simulink model "Quadcopter_nonlinear"  (R2023a)
settings: Solver=ode4  StartTime=0.0  StopTime=0.2  FixedStep=0.02  RelTol=1e-3
values from neighbouring files (symbols this model uses):
  b = 1.10794e-5    (= 1.10794e-05)    [QuadParameter.m]
  d = 3.2e-6    (= 3.2e-06)    [QuadParameter.m]
  d_cg = 0.295    [QuadParameter.m]
  Gamma1 = 4.98954110218396e-06    (= 4.98954110218e-06)    [final_PS.m]
  Gamma10 = -1.44562619785504e-05    (= -1.44562619786e-05)    [final_PS.m]
  Gamma11 = 24.4566929368231    (= 24.4566929368)    [final_PS.m]
  Gamma2 = 0.00290613207976024    (= 0.00290613207976)    [final_PS.m]
  Gamma3 = 42.1805100768496    (= 42.1805100768)    [final_PS.m]
  Gamma4 = 0.000237183411278011    (= 0.000237183411278)    [final_PS.m]
  Gamma5 = -0.00234577516229748    (= -0.0023457751623)    [final_PS.m]
  Gamma6 = 2.52935414320957    (= 2.52935414321)    [final_PS.m]
  Gamma7 = 0.000224057181768728    (= 0.000224057181769)    [final_PS.m]
  Gamma8 = 18.4688604256806    (= 18.4688604257)    [final_PS.m]
  Gamma9 = 0.00216966508125569    (= 0.00216966508126)    [final_PS.m]
  init_I = data_I(1, :)    [PS_I.m]
  init_II = data_II(1, :)    [PS_II.m]
  init_III = data_III(1, :)    [PS_III.m]
  init_IV = data_IV(1, :)    [PS_IV.m]
  init_IX = data_IX(1, :)    [PS_IX.m]
  init_V = data_V(1, :)    [PS_V.m]
  init_VI = data_VI(1, :)    [PS_VI.m]
  Omega_I = Omega(1, :)    [PS_I.m]
  Omega_II = Omega(1, :)    [PS_II.m]
  Omega_III = Omega(1, :)    [PS_III.m]
  Omega_IV = Omega(1, :)    [PS_IV.m]
  Omega_IX = Omega(1, :)    [PS_IX.m]
  Omega_V = Omega(1, :)    [PS_V.m]
  Omega_VI = Omega(1, :)    [PS_VI.m]
  Omega_VII = Omega(1, :)    [PS_VII.m]
  Omega_VIII = Omega(1, :)    [PS_VIII.m]
  Omega_X = Omega(1, :)    [PS_X.m]
undefined symbols (not defined in the file or in its folder): init_VII, init_VIII, init_X
(part 3 of 3)

== system Quadcopter_nonlinear/Quadcopter 3DOF Nonlinear System8/Quad System1/Quad System/dot(x1)/Subsystem1 ==
  X : Inport
  Demux : Demux  Outputs=6
  Terminator{,2..5} (5 alike) : Terminator
  x4 : Outport
  wires:
  Demux/6 -> Terminator5/1  "x6"
  X/1 -> Demux/1
  Demux/3 -> Terminator/1  "x3"
  Demux/1 -> Terminator4/1  "x1"
  Demux/2 -> Terminator2/1  "x2"
  Demux/5 -> Terminator3/1  "x5"
  Demux/4 -> x4/1  "x4"

== system Quadcopter_nonlinear/Quadcopter 3DOF Nonlinear System8/Quad System1/Quad System/dot(x2)/1 ==
  X : Inport
  Demux : Demux  Outputs=6
  Subsystem : Subsystem
  Terminator{,1..3} (4 alike) : Terminator
  x5cos(x1) : Outport
  wires:
  Demux/4 -> Terminator1/1  "x4"
  X/1 -> Demux/1  "x"
  Demux/1 -> Subsystem/1(x1)  "x1"
  Demux/3 -> Terminator/1  "x3"
  Demux/6 -> Terminator2/1  "x6"
  Demux/5 -> Subsystem/2(x5)  "x5"
  Subsystem/1(Out1) -> x5cos(x1)/1
  Demux/2 -> Terminator3/1  "x2"

== system Quadcopter_nonlinear/Quadcopter 3DOF Nonlinear System8/Quad System1/Quad System/dot(x2)/Subsystem ==
  X : Inport
  Demux : Demux  Outputs=6
  Subsystem1 : Subsystem
  Terminator{,1..3} (4 alike) : Terminator
  x6sin(x1) : Outport
  wires:
  Demux/1 -> Subsystem1/1(x1)  "x1"
  Demux/3 -> Terminator/1  "x3"
  Demux/4 -> Terminator1/1  "x4"
  Demux/5 -> Terminator3/1  "x5"
  Demux/6 -> Subsystem1/2(x6)  "x6"
  Subsystem1/1(Out1) -> x6sin(x1)/1  "x6sin(x1)"
  X/1 -> Demux/1  "X"
  Demux/2 -> Terminator2/1  "x2"

== system Quadcopter_nonlinear/Quadcopter 3DOF Nonlinear System8/Quad System1/Quad System/dot(x3)/1 ==
  X : Inport
  Demux : Demux  Outputs=6
  Subsystem : Subsystem
  Terminator{,1..3} (4 alike) : Terminator
  x5sin(x1) : Outport
  wires:
  Demux/4 -> Terminator1/1  "x4"
  X/1 -> Demux/1  "x"
  Demux/1 -> Subsystem/1(x1)  "x1"
  Demux/3 -> Terminator/1  "x3"
  Demux/6 -> Terminator2/1  "x6"
  Demux/5 -> Subsystem/2(x5)  "x5"
  Subsystem/1(x5sin(x1)) -> x5sin(x1)/1
  Demux/2 -> Terminator3/1  "x2"

== system Quadcopter_nonlinear/Quadcopter 3DOF Nonlinear System8/Quad System1/Quad System/dot(x3)/Subsystem ==
  X : Inport
  Demux : Demux  Outputs=6
  Subsystem1 : Subsystem
  Terminator{,1..3} (4 alike) : Terminator
  x6cos(x1) : Outport
  wires:
  Demux/1 -> Subsystem1/1(x1)  "x1"
  Demux/3 -> Terminator/1  "x3"
  Demux/4 -> Terminator1/1  "x4"
  Demux/5 -> Terminator3/1  "x5"
  Demux/6 -> Subsystem1/2(x6)  "x6"
  Subsystem1/1(Out1) -> x6cos(x1)/1  "x6cos(x1)"
  X/1 -> Demux/1  "X"
  Demux/2 -> Terminator2/1  "x2"

== system Quadcopter_nonlinear/Quadcopter 3DOF Nonlinear System8/Quad System1/Quad System/dot(x3)/Subsystem1 ==
  X : Inport
  Demux : Demux  Outputs=6
  Sec : Subsystem
  Terminator{,1..4} (5 alike) : Terminator
  sec(x2) : Outport
  wires:
  Demux/3 -> Terminator/1  "x3"
  Demux/4 -> Terminator1/1  "x4"
  Demux/5 -> Terminator3/1  "x5"
  X/1 -> Demux/1  "X"
  Demux/1 -> Terminator2/1  "x1"
  Demux/6 -> Terminator4/1  "x6"
  Demux/2 -> Sec/1(x2)  "x2"
  Sec/1(Sec(x2)) -> sec(x2)/1

== system Quadcopter_nonlinear/Quadcopter 3DOF Nonlinear System9/Quad System1/Quad System/dot(x1)/1 ==
  X : Inport
  Demux : Demux  Outputs=6
  Subsystem : Subsystem
  Terminator : Terminator
  Terminator1 : Terminator
  Terminator2 : Terminator
  x5sin(x1)tan(x2) : Outport
  wires:
  Demux/2 -> Subsystem/2(x2)  "x2"
  Demux/4 -> Terminator1/1  "x4"
  X/1 -> Demux/1  "x"
  Demux/1 -> Subsystem/1(x1)  "x1"
  Demux/3 -> Terminator/1  "x3"
  Demux/6 -> Terminator2/1  "x6"
  Demux/5 -> Subsystem/3(x5)  "x5"
  Subsystem/1(x5sin(x1)tan(x2)) -> x5sin(x1)tan(x2)/1

== system Quadcopter_nonlinear/Quadcopter 3DOF Nonlinear System9/Quad System1/Quad System/dot(x1)/Subsystem ==
  X : Inport
  Demux : Demux  Outputs=6
  Subsystem1 : Subsystem
  Terminator : Terminator
  Terminator1 : Terminator
  Terminator3 : Terminator
  x6cos(x1)tan(x2) : Outport
  wires:
  Demux/1 -> Subsystem1/1(x1)  "x1"
  Demux/3 -> Terminator/1  "x3"
  Demux/4 -> Terminator1/1  "x4"
  Demux/5 -> Terminator3/1  "x5"
  Demux/6 -> Subsystem1/3(x6)  "x6"
  Subsystem1/1(x6cos(x1)tan(x2)) -> x6cos(x1)tan(x2)/1  "x6cos(x1)tan(x2)"
  X/1 -> Demux/1  "X"
  Demux/2 -> Subsystem1/2(x2)  "x2"

== system Quadcopter_nonlinear/Quadcopter 3DOF Nonlinear System9/Quad System1/Quad System/dot(x1)/Subsystem1 ==
  X : Inport
  Demux : Demux  Outputs=6
  Terminator{,2..5} (5 alike) : Terminator
  x4 : Outport
  wires:
  Demux/6 -> Terminator5/1  "x6"
  X/1 -> Demux/1
  Demux/3 -> Terminator/1  "x3"
  Demux/1 -> Terminator4/1  "x1"
  Demux/2 -> Terminator2/1  "x2"
  Demux/5 -> Terminator3/1  "x5"
  Demux/4 -> x4/1  "x4"

== system Quadcopter_nonlinear/Quadcopter 3DOF Nonlinear System9/Quad System1/Quad System/dot(x2)/1 ==
  X : Inport
  Demux : Demux  Outputs=6
  Subsystem : Subsystem
  Terminator{,1..3} (4 alike) : Terminator
  x5cos(x1) : Outport
  wires:
  Demux/4 -> Terminator1/1  "x4"
  X/1 -> Demux/1  "x"
  Demux/1 -> Subsystem/1(x1)  "x1"
  Demux/3 -> Terminator/1  "x3"
  Demux/6 -> Terminator2/1  "x6"
  Demux/5 -> Subsystem/2(x5)  "x5"
  Subsystem/1(Out1) -> x5cos(x1)/1
  Demux/2 -> Terminator3/1  "x2"

== system Quadcopter_nonlinear/Quadcopter 3DOF Nonlinear System9/Quad System1/Quad System/dot(x2)/Subsystem ==
  X : Inport
  Demux : Demux  Outputs=6
  Subsystem1 : Subsystem
  Terminator{,1..3} (4 alike) : Terminator
  x6sin(x1) : Outport
  wires:
  Demux/1 -> Subsystem1/1(x1)  "x1"
  Demux/3 -> Terminator/1  "x3"
  Demux/4 -> Terminator1/1  "x4"
  Demux/5 -> Terminator3/1  "x5"
  Demux/6 -> Subsystem1/2(x6)  "x6"
  Subsystem1/1(Out1) -> x6sin(x1)/1  "x6sin(x1)"
  X/1 -> Demux/1  "X"
  Demux/2 -> Terminator2/1  "x2"

== system Quadcopter_nonlinear/Quadcopter 3DOF Nonlinear System9/Quad System1/Quad System/dot(x3)/1 ==
  X : Inport
  Demux : Demux  Outputs=6
  Subsystem : Subsystem
  Terminator{,1..3} (4 alike) : Terminator
  x5sin(x1) : Outport
  wires:
  Demux/4 -> Terminator1/1  "x4"
  X/1 -> Demux/1  "x"
  Demux/1 -> Subsystem/1(x1)  "x1"
  Demux/3 -> Terminator/1  "x3"
  Demux/6 -> Terminator2/1  "x6"
  Demux/5 -> Subsystem/2(x5)  "x5"
  Subsystem/1(x5sin(x1)) -> x5sin(x1)/1
  Demux/2 -> Terminator3/1  "x2"

== system Quadcopter_nonlinear/Quadcopter 3DOF Nonlinear System9/Quad System1/Quad System/dot(x3)/Subsystem ==
  X : Inport
  Demux : Demux  Outputs=6
  Subsystem1 : Subsystem
  Terminator{,1..3} (4 alike) : Terminator
  x6cos(x1) : Outport
  wires:
  Demux/1 -> Subsystem1/1(x1)  "x1"
  Demux/3 -> Terminator/1  "x3"
  Demux/4 -> Terminator1/1  "x4"
  Demux/5 -> Terminator3/1  "x5"
  Demux/6 -> Subsystem1/2(x6)  "x6"
  Subsystem1/1(Out1) -> x6cos(x1)/1  "x6cos(x1)"
  X/1 -> Demux/1  "X"
  Demux/2 -> Terminator2/1  "x2"

== system Quadcopter_nonlinear/Quadcopter 3DOF Nonlinear System9/Quad System1/Quad System/dot(x3)/Subsystem1 ==
  X : Inport
  Demux : Demux  Outputs=6
  Sec : Subsystem
  Terminator{,1..4} (5 alike) : Terminator
  sec(x2) : Outport
  wires:
  Demux/3 -> Terminator/1  "x3"
  Demux/4 -> Terminator1/1  "x4"
  Demux/5 -> Terminator3/1  "x5"
  X/1 -> Demux/1  "X"
  Demux/1 -> Terminator2/1  "x1"
  Demux/6 -> Terminator4/1  "x6"
  Demux/2 -> Sec/1(x2)  "x2"
  Sec/1(Sec(x2)) -> sec(x2)/1

== system Quadcopter_nonlinear/Quadcopter 3DOF Nonlinear System/Quad System1/Quad System/dot(x1)/1/Subsystem ==
  x1 : Inport
  x2 : Inport  Port=2
  x5 : Inport  Port=3
  Product : Product  Inputs=3
  Sin : Trigonometry
  Tan : Trigonometry  Operator=tan
  x5sin(x1)tan(x2) : Outport
  wires:
  Sin/1 -> Product/1
  x5/1 -> Product/3
  Product/1 -> x5sin(x1)tan(x2)/1
  x1/1 -> Sin/1
  x2/1 -> Tan/1
  Tan/1 -> Product/2

== system Quadcopter_nonlinear/Quadcopter 3DOF Nonlinear System/Quad System1/Quad System/dot(x1)/Subsystem/Subsystem1 ==
  x1 : Inport
  x2 : Inport  Port=2
  x6 : Inport  Port=3
  Cos : Trigonometry  Operator=cos
  Product1 : Product  Inputs=3
  Tan : Trigonometry  Operator=tan
  x6cos(x1)tan(x2) : Outport
  wires:
  x6/1 -> Product1/3
  x1/1 -> Cos/1
  Cos/1 -> Product1/1
  x2/1 -> Tan/1
  Product1/1 -> x6cos(x1)tan(x2)/1
  Tan/1 -> Product1/2

== system Quadcopter_nonlinear/Quadcopter 3DOF Nonlinear System/Quad System1/Quad System/dot(x2)/1/Subsystem ==
  x1 : Inport
  x5 : Inport  Port=2
  Cos : Trigonometry  Operator=cos
  Product : Product
  Out1 : Outport
  wires:
  Cos/1 -> Product/1
  Product/1 -> Out1/1
  x1/1 -> Cos/1
  x5/1 -> Product/2

== system Quadcopter_nonlinear/Quadcopter 3DOF Nonlinear System/Quad System1/Quad System/dot(x2)/Subsystem/Subsystem1 ==
  x1 : Inport
  x6 : Inport  Port=2
  Product1 : Product
  Sin : Trigonometry
  Out1 : Outport
  wires:
  x6/1 -> Product1/2
  x1/1 -> Sin/1
  Sin/1 -> Product1/1
  Product1/1 -> Out1/1

== system Quadcopter_nonlinear/Quadcopter 3DOF Nonlinear System/Quad System1/Quad System/dot(x3)/1/Subsystem ==
  x1 : Inport
  x5 : Inport  Port=2
  Product : Product
  Sin : Trigonometry
  x5sin(x1) : Outport
  wires:
  Sin/1 -> Product/1
  Product/1 -> x5sin(x1)/1
  x1/1 -> Sin/1
  x5/1 -> Product/2

== system Quadcopter_nonlinear/Quadcopter 3DOF Nonlinear System/Quad System1/Quad System/dot(x3)/Subsystem/Subsystem1 ==
  x1 : Inport
  x6 : Inport  Port=2
  Cos : Trigonometry  Operator=cos
  Product1 : Product
  Out1 : Outport
  wires:
  x6/1 -> Product1/2
  x1/1 -> Cos/1
  Cos/1 -> Product1/1
  Product1/1 -> Out1/1

== system Quadcopter_nonlinear/Quadcopter 3DOF Nonlinear System/Quad System1/Quad System/dot(x3)/Subsystem1/Sec ==
  x2 : Inport
  Constant : Constant
  Cos : Trigonometry  Operator=cos
  Divide : Product  Inputs=*/
  Sec(x2) : Outport
  wires:
  Constant/1 -> Divide/1
  Cos/1 -> Divide/2
  Divide/1 -> Sec(x2)/1
  x2/1 -> Cos/1

== system Quadcopter_nonlinear/Quadcopter 3DOF Nonlinear System1/Quad System1/Quad System/dot(x1)/1/Subsystem ==
  x1 : Inport
  x2 : Inport  Port=2
  x5 : Inport  Port=3
  Product : Product  Inputs=3
  Sin : Trigonometry
  Tan : Trigonometry  Operator=tan
  x5sin(x1)tan(x2) : Outport
  wires:
  Sin/1 -> Product/1
  x5/1 -> Product/3
  Product/1 -> x5sin(x1)tan(x2)/1
  x1/1 -> Sin/1
  x2/1 -> Tan/1
  Tan/1 -> Product/2

== system Quadcopter_nonlinear/Quadcopter 3DOF Nonlinear System1/Quad System1/Quad System/dot(x1)/Subsystem/Subsystem1 ==
  x1 : Inport
  x2 : Inport  Port=2
  x6 : Inport  Port=3
  Cos : Trigonometry  Operator=cos
  Product1 : Product  Inputs=3
  Tan : Trigonometry  Operator=tan
  x6cos(x1)tan(x2) : Outport
  wires:
  x6/1 -> Product1/3
  x1/1 -> Cos/1
  Cos/1 -> Product1/1
  x2/1 -> Tan/1
  Product1/1 -> x6cos(x1)tan(x2)/1
  Tan/1 -> Product1/2

== system Quadcopter_nonlinear/Quadcopter 3DOF Nonlinear System1/Quad System1/Quad System/dot(x2)/1/Subsystem ==
  x1 : Inport
  x5 : Inport  Port=2
  Cos : Trigonometry  Operator=cos
  Product : Product
  Out1 : Outport
  wires:
  Cos/1 -> Product/1
  Product/1 -> Out1/1
  x1/1 -> Cos/1
  x5/1 -> Product/2

== system Quadcopter_nonlinear/Quadcopter 3DOF Nonlinear System1/Quad System1/Quad System/dot(x2)/Subsystem/Subsystem1 ==
  x1 : Inport
  x6 : Inport  Port=2
  Product1 : Product
  Sin : Trigonometry
  Out1 : Outport
  wires:
  x6/1 -> Product1/2
  x1/1 -> Sin/1
  Sin/1 -> Product1/1
  Product1/1 -> Out1/1

== system Quadcopter_nonlinear/Quadcopter 3DOF Nonlinear System1/Quad System1/Quad System/dot(x3)/1/Subsystem ==
  x1 : Inport
  x5 : Inport  Port=2
  Product : Product
  Sin : Trigonometry
  x5sin(x1) : Outport
  wires:
  Sin/1 -> Product/1
  Product/1 -> x5sin(x1)/1
  x1/1 -> Sin/1
  x5/1 -> Product/2

== system Quadcopter_nonlinear/Quadcopter 3DOF Nonlinear System1/Quad System1/Quad System/dot(x3)/Subsystem/Subsystem1 ==
  x1 : Inport
  x6 : Inport  Port=2
  Cos : Trigonometry  Operator=cos
  Product1 : Product
  Out1 : Outport
  wires:
  x6/1 -> Product1/2
  x1/1 -> Cos/1
  Cos/1 -> Product1/1
  Product1/1 -> Out1/1

== system Quadcopter_nonlinear/Quadcopter 3DOF Nonlinear System1/Quad System1/Quad System/dot(x3)/Subsystem1/Sec ==
  x2 : Inport
  Constant : Constant
  Cos : Trigonometry  Operator=cos
  Divide : Product  Inputs=*/
  Sec(x2) : Outport
  wires:
  Constant/1 -> Divide/1
  Cos/1 -> Divide/2
  Divide/1 -> Sec(x2)/1
  x2/1 -> Cos/1

== system Quadcopter_nonlinear/Quadcopter 3DOF Nonlinear System2/Quad System1/Quad System/dot(x1)/1/Subsystem ==
  x1 : Inport
  x2 : Inport  Port=2
  x5 : Inport  Port=3
  Product : Product  Inputs=3
  Sin : Trigonometry
  Tan : Trigonometry  Operator=tan
  x5sin(x1)tan(x2) : Outport
  wires:
  Sin/1 -> Product/1
  x5/1 -> Product/3
  Product/1 -> x5sin(x1)tan(x2)/1
  x1/1 -> Sin/1
  x2/1 -> Tan/1
  Tan/1 -> Product/2

== system Quadcopter_nonlinear/Quadcopter 3DOF Nonlinear System2/Quad System1/Quad System/dot(x1)/Subsystem/Subsystem1 ==
  x1 : Inport
  x2 : Inport  Port=2
  x6 : Inport  Port=3
  Cos : Trigonometry  Operator=cos
  Product1 : Product  Inputs=3
  Tan : Trigonometry  Operator=tan
  x6cos(x1)tan(x2) : Outport
  wires:
  x6/1 -> Product1/3
  x1/1 -> Cos/1
  Cos/1 -> Product1/1
  x2/1 -> Tan/1
  Product1/1 -> x6cos(x1)tan(x2)/1
  Tan/1 -> Product1/2

== system Quadcopter_nonlinear/Quadcopter 3DOF Nonlinear System2/Quad System1/Quad System/dot(x2)/1/Subsystem ==
  x1 : Inport
  x5 : Inport  Port=2
  Cos : Trigonometry  Operator=cos
  Product : Product
  Out1 : Outport
  wires:
  Cos/1 -> Product/1
  Product/1 -> Out1/1
  x1/1 -> Cos/1
  x5/1 -> Product/2

== system Quadcopter_nonlinear/Quadcopter 3DOF Nonlinear System2/Quad System1/Quad System/dot(x2)/Subsystem/Subsystem1 ==
  x1 : Inport
  x6 : Inport  Port=2
  Product1 : Product
  Sin : Trigonometry
  Out1 : Outport
  wires:
  x6/1 -> Product1/2
  x1/1 -> Sin/1
  Sin/1 -> Product1/1
  Product1/1 -> Out1/1

== system Quadcopter_nonlinear/Quadcopter 3DOF Nonlinear System2/Quad System1/Quad System/dot(x3)/1/Subsystem ==
  x1 : Inport
  x5 : Inport  Port=2
  Product : Product
  Sin : Trigonometry
  x5sin(x1) : Outport
  wires:
  Sin/1 -> Product/1
  Product/1 -> x5sin(x1)/1
  x1/1 -> Sin/1
  x5/1 -> Product/2

== system Quadcopter_nonlinear/Quadcopter 3DOF Nonlinear System2/Quad System1/Quad System/dot(x3)/Subsystem/Subsystem1 ==
  x1 : Inport
  x6 : Inport  Port=2
  Cos : Trigonometry  Operator=cos
  Product1 : Product
  Out1 : Outport
  wires:
  x6/1 -> Product1/2
  x1/1 -> Cos/1
  Cos/1 -> Product1/1
  Product1/1 -> Out1/1

== system Quadcopter_nonlinear/Quadcopter 3DOF Nonlinear System2/Quad System1/Quad System/dot(x3)/Subsystem1/Sec ==
  x2 : Inport
  Constant : Constant
  Cos : Trigonometry  Operator=cos
  Divide : Product  Inputs=*/
  Sec(x2) : Outport
  wires:
  Constant/1 -> Divide/1
  Cos/1 -> Divide/2
  Divide/1 -> Sec(x2)/1
  x2/1 -> Cos/1

== system Quadcopter_nonlinear/Quadcopter 3DOF Nonlinear System3/Quad System1/Quad System/dot(x1)/1/Subsystem ==
  x1 : Inport
  x2 : Inport  Port=2
  x5 : Inport  Port=3
  Product : Product  Inputs=3
  Sin : Trigonometry
  Tan : Trigonometry  Operator=tan
  x5sin(x1)tan(x2) : Outport
  wires:
  Sin/1 -> Product/1
  x5/1 -> Product/3
  Product/1 -> x5sin(x1)tan(x2)/1
  x1/1 -> Sin/1
  x2/1 -> Tan/1
  Tan/1 -> Product/2

== system Quadcopter_nonlinear/Quadcopter 3DOF Nonlinear System3/Quad System1/Quad System/dot(x1)/Subsystem/Subsystem1 ==
  x1 : Inport
  x2 : Inport  Port=2
  x6 : Inport  Port=3
  Cos : Trigonometry  Operator=cos
  Product1 : Product  Inputs=3
  Tan : Trigonometry  Operator=tan
  x6cos(x1)tan(x2) : Outport
  wires:
  x6/1 -> Product1/3
  x1/1 -> Cos/1
  Cos/1 -> Product1/1
  x2/1 -> Tan/1
  Product1/1 -> x6cos(x1)tan(x2)/1
  Tan/1 -> Product1/2

== system Quadcopter_nonlinear/Quadcopter 3DOF Nonlinear System3/Quad System1/Quad System/dot(x2)/1/Subsystem ==
  x1 : Inport
  x5 : Inport  Port=2
  Cos : Trigonometry  Operator=cos
  Product : Product
  Out1 : Outport
  wires:
  Cos/1 -> Product/1
  Product/1 -> Out1/1
  x1/1 -> Cos/1
  x5/1 -> Product/2

== system Quadcopter_nonlinear/Quadcopter 3DOF Nonlinear System3/Quad System1/Quad System/dot(x2)/Subsystem/Subsystem1 ==
  x1 : Inport
  x6 : Inport  Port=2
  Product1 : Product
  Sin : Trigonometry
  Out1 : Outport
  wires:
  x6/1 -> Product1/2
  x1/1 -> Sin/1
  Sin/1 -> Product1/1
  Product1/1 -> Out1/1

== system Quadcopter_nonlinear/Quadcopter 3DOF Nonlinear System3/Quad System1/Quad System/dot(x3)/1/Subsystem ==
  x1 : Inport
  x5 : Inport  Port=2
  Product : Product
  Sin : Trigonometry
  x5sin(x1) : Outport
  wires:
  Sin/1 -> Product/1
  Product/1 -> x5sin(x1)/1
  x1/1 -> Sin/1
  x5/1 -> Product/2

== system Quadcopter_nonlinear/Quadcopter 3DOF Nonlinear System3/Quad System1/Quad System/dot(x3)/Subsystem/Subsystem1 ==
  x1 : Inport
  x6 : Inport  Port=2
  Cos : Trigonometry  Operator=cos
  Product1 : Product
  Out1 : Outport
  wires:
  x6/1 -> Product1/2
  x1/1 -> Cos/1
  Cos/1 -> Product1/1
  Product1/1 -> Out1/1

== system Quadcopter_nonlinear/Quadcopter 3DOF Nonlinear System3/Quad System1/Quad System/dot(x3)/Subsystem1/Sec ==
  x2 : Inport
  Constant : Constant
  Cos : Trigonometry  Operator=cos
  Divide : Product  Inputs=*/
  Sec(x2) : Outport
  wires:
  Constant/1 -> Divide/1
  Cos/1 -> Divide/2
  Divide/1 -> Sec(x2)/1
  x2/1 -> Cos/1

== system Quadcopter_nonlinear/Quadcopter 3DOF Nonlinear System4/Quad System1/Quad System/dot(x1)/1/Subsystem ==
  x1 : Inport
  x2 : Inport  Port=2
  x5 : Inport  Port=3
  Product : Product  Inputs=3
  Sin : Trigonometry
  Tan : Trigonometry  Operator=tan
  x5sin(x1)tan(x2) : Outport
  wires:
  Sin/1 -> Product/1
  x5/1 -> Product/3
  Product/1 -> x5sin(x1)tan(x2)/1
  x1/1 -> Sin/1
  x2/1 -> Tan/1
  Tan/1 -> Product/2

== system Quadcopter_nonlinear/Quadcopter 3DOF Nonlinear System4/Quad System1/Quad System/dot(x1)/Subsystem/Subsystem1 ==
  x1 : Inport
  x2 : Inport  Port=2
  x6 : Inport  Port=3
  Cos : Trigonometry  Operator=cos
  Product1 : Product  Inputs=3
  Tan : Trigonometry  Operator=tan
  x6cos(x1)tan(x2) : Outport
  wires:
  x6/1 -> Product1/3
  x1/1 -> Cos/1
  Cos/1 -> Product1/1
  x2/1 -> Tan/1
  Product1/1 -> x6cos(x1)tan(x2)/1
  Tan/1 -> Product1/2

== system Quadcopter_nonlinear/Quadcopter 3DOF Nonlinear System4/Quad System1/Quad System/dot(x2)/1/Subsystem ==
  x1 : Inport
  x5 : Inport  Port=2
  Cos : Trigonometry  Operator=cos
  Product : Product
  Out1 : Outport
  wires:
  Cos/1 -> Product/1
  Product/1 -> Out1/1
  x1/1 -> Cos/1
  x5/1 -> Product/2

== system Quadcopter_nonlinear/Quadcopter 3DOF Nonlinear System4/Quad System1/Quad System/dot(x2)/Subsystem/Subsystem1 ==
  x1 : Inport
  x6 : Inport  Port=2
  Product1 : Product
  Sin : Trigonometry
  Out1 : Outport
  wires:
  x6/1 -> Product1/2
  x1/1 -> Sin/1
  Sin/1 -> Product1/1
  Product1/1 -> Out1/1

== system Quadcopter_nonlinear/Quadcopter 3DOF Nonlinear System4/Quad System1/Quad System/dot(x3)/1/Subsystem ==
  x1 : Inport
  x5 : Inport  Port=2
  Product : Product
  Sin : Trigonometry
  x5sin(x1) : Outport
  wires:
  Sin/1 -> Product/1
  Product/1 -> x5sin(x1)/1
  x1/1 -> Sin/1
  x5/1 -> Product/2

== system Quadcopter_nonlinear/Quadcopter 3DOF Nonlinear System4/Quad System1/Quad System/dot(x3)/Subsystem/Subsystem1 ==
  x1 : Inport
  x6 : Inport  Port=2
  Cos : Trigonometry  Operator=cos
  Product1 : Product
  Out1 : Outport
  wires:
  x6/1 -> Product1/2
  x1/1 -> Cos/1
  Cos/1 -> Product1/1
  Product1/1 -> Out1/1

== system Quadcopter_nonlinear/Quadcopter 3DOF Nonlinear System4/Quad System1/Quad System/dot(x3)/Subsystem1/Sec ==
  x2 : Inport
  Constant : Constant
  Cos : Trigonometry  Operator=cos
  Divide : Product  Inputs=*/
  Sec(x2) : Outport
  wires:
  Constant/1 -> Divide/1
  Cos/1 -> Divide/2
  Divide/1 -> Sec(x2)/1
  x2/1 -> Cos/1

== system Quadcopter_nonlinear/Quadcopter 3DOF Nonlinear System5/Quad System1/Quad System/dot(x1)/1/Subsystem ==
  x1 : Inport
  x2 : Inport  Port=2
  x5 : Inport  Port=3
  Product : Product  Inputs=3
  Sin : Trigonometry
  Tan : Trigonometry  Operator=tan
  x5sin(x1)tan(x2) : Outport
  wires:
  Sin/1 -> Product/1
  x5/1 -> Product/3
  Product/1 -> x5sin(x1)tan(x2)/1
  x1/1 -> Sin/1
  x2/1 -> Tan/1
  Tan/1 -> Product/2

== system Quadcopter_nonlinear/Quadcopter 3DOF Nonlinear System5/Quad System1/Quad System/dot(x1)/Subsystem/Subsystem1 ==
  x1 : Inport
  x2 : Inport  Port=2
  x6 : Inport  Port=3
  Cos : Trigonometry  Operator=cos
  Product1 : Product  Inputs=3
  Tan : Trigonometry  Operator=tan
  x6cos(x1)tan(x2) : Outport
  wires:
  x6/1 -> Product1/3
  x1/1 -> Cos/1
  Cos/1 -> Product1/1
  x2/1 -> Tan/1
  Product1/1 -> x6cos(x1)tan(x2)/1
  Tan/1 -> Product1/2

== system Quadcopter_nonlinear/Quadcopter 3DOF Nonlinear System5/Quad System1/Quad System/dot(x2)/1/Subsystem ==
  x1 : Inport
  x5 : Inport  Port=2
  Cos : Trigonometry  Operator=cos
  Product : Product
  Out1 : Outport
  wires:
  Cos/1 -> Product/1
  Product/1 -> Out1/1
  x1/1 -> Cos/1
  x5/1 -> Product/2

== system Quadcopter_nonlinear/Quadcopter 3DOF Nonlinear System5/Quad System1/Quad System/dot(x2)/Subsystem/Subsystem1 ==
  x1 : Inport
  x6 : Inport  Port=2
  Product1 : Product
  Sin : Trigonometry
  Out1 : Outport
  wires:
  x6/1 -> Product1/2
  x1/1 -> Sin/1
  Sin/1 -> Product1/1
  Product1/1 -> Out1/1

== system Quadcopter_nonlinear/Quadcopter 3DOF Nonlinear System5/Quad System1/Quad System/dot(x3)/1/Subsystem ==
  x1 : Inport
  x5 : Inport  Port=2
  Product : Product
  Sin : Trigonometry
  x5sin(x1) : Outport
  wires:
  Sin/1 -> Product/1
  Product/1 -> x5sin(x1)/1
  x1/1 -> Sin/1
  x5/1 -> Product/2

== system Quadcopter_nonlinear/Quadcopter 3DOF Nonlinear System5/Quad System1/Quad System/dot(x3)/Subsystem/Subsystem1 ==
  x1 : Inport
  x6 : Inport  Port=2
  Cos : Trigonometry  Operator=cos
  Product1 : Product
  Out1 : Outport
  wires:
  x6/1 -> Product1/2
  x1/1 -> Cos/1
  Cos/1 -> Product1/1
  Product1/1 -> Out1/1

== system Quadcopter_nonlinear/Quadcopter 3DOF Nonlinear System5/Quad System1/Quad System/dot(x3)/Subsystem1/Sec ==
  x2 : Inport
  Constant : Constant
  Cos : Trigonometry  Operator=cos
  Divide : Product  Inputs=*/
  Sec(x2) : Outport
  wires:
  Constant/1 -> Divide/1
  Cos/1 -> Divide/2
  Divide/1 -> Sec(x2)/1
  x2/1 -> Cos/1

== system Quadcopter_nonlinear/Quadcopter 3DOF Nonlinear System6/Quad System1/Quad System/dot(x1)/1/Subsystem ==
  x1 : Inport
  x2 : Inport  Port=2
  x5 : Inport  Port=3
  Product : Product  Inputs=3
  Sin : Trigonometry
  Tan : Trigonometry  Operator=tan
  x5sin(x1)tan(x2) : Outport
  wires:
  Sin/1 -> Product/1
  x5/1 -> Product/3
  Product/1 -> x5sin(x1)tan(x2)/1
  x1/1 -> Sin/1
  x2/1 -> Tan/1
  Tan/1 -> Product/2

== system Quadcopter_nonlinear/Quadcopter 3DOF Nonlinear System6/Quad System1/Quad System/dot(x1)/Subsystem/Subsystem1 ==
  x1 : Inport
  x2 : Inport  Port=2
  x6 : Inport  Port=3
  Cos : Trigonometry  Operator=cos
  Product1 : Product  Inputs=3
  Tan : Trigonometry  Operator=tan
  x6cos(x1)tan(x2) : Outport
  wires:
  x6/1 -> Product1/3
  x1/1 -> Cos/1
  Cos/1 -> Product1/1
  x2/1 -> Tan/1
  Product1/1 -> x6cos(x1)tan(x2)/1
  Tan/1 -> Product1/2

== system Quadcopter_nonlinear/Quadcopter 3DOF Nonlinear System6/Quad System1/Quad System/dot(x2)/1/Subsystem ==
  x1 : Inport
  x5 : Inport  Port=2
  Cos : Trigonometry  Operator=cos
  Product : Product
  Out1 : Outport
  wires:
  Cos/1 -> Product/1
  Product/1 -> Out1/1
  x1/1 -> Cos/1
  x5/1 -> Product/2

== system Quadcopter_nonlinear/Quadcopter 3DOF Nonlinear System6/Quad System1/Quad System/dot(x2)/Subsystem/Subsystem1 ==
  x1 : Inport
  x6 : Inport  Port=2
  Product1 : Product
  Sin : Trigonometry
  Out1 : Outport
  wires:
  x6/1 -> Product1/2
  x1/1 -> Sin/1
  Sin/1 -> Product1/1
  Product1/1 -> Out1/1

== system Quadcopter_nonlinear/Quadcopter 3DOF Nonlinear System6/Quad System1/Quad System/dot(x3)/1/Subsystem ==
  x1 : Inport
  x5 : Inport  Port=2
  Product : Product
  Sin : Trigonometry
  x5sin(x1) : Outport
  wires:
  Sin/1 -> Product/1
  Product/1 -> x5sin(x1)/1
  x1/1 -> Sin/1
  x5/1 -> Product/2

== system Quadcopter_nonlinear/Quadcopter 3DOF Nonlinear System6/Quad System1/Quad System/dot(x3)/Subsystem/Subsystem1 ==
  x1 : Inport
  x6 : Inport  Port=2
  Cos : Trigonometry  Operator=cos
  Product1 : Product
  Out1 : Outport
  wires:
  x6/1 -> Product1/2
  x1/1 -> Cos/1
  Cos/1 -> Product1/1
  Product1/1 -> Out1/1

== system Quadcopter_nonlinear/Quadcopter 3DOF Nonlinear System6/Quad System1/Quad System/dot(x3)/Subsystem1/Sec ==
  x2 : Inport
  Constant : Constant
  Cos : Trigonometry  Operator=cos
  Divide : Product  Inputs=*/
  Sec(x2) : Outport
  wires:
  Constant/1 -> Divide/1
  Cos/1 -> Divide/2
  Divide/1 -> Sec(x2)/1
  x2/1 -> Cos/1

== system Quadcopter_nonlinear/Quadcopter 3DOF Nonlinear System7/Quad System1/Quad System/dot(x1)/1/Subsystem ==
  x1 : Inport
  x2 : Inport  Port=2
  x5 : Inport  Port=3
  Product : Product  Inputs=3
  Sin : Trigonometry
  Tan : Trigonometry  Operator=tan
  x5sin(x1)tan(x2) : Outport
  wires:
  Sin/1 -> Product/1
  x5/1 -> Product/3
  Product/1 -> x5sin(x1)tan(x2)/1
  x1/1 -> Sin/1
  x2/1 -> Tan/1
  Tan/1 -> Product/2

== system Quadcopter_nonlinear/Quadcopter 3DOF Nonlinear System7/Quad System1/Quad System/dot(x1)/Subsystem/Subsystem1 ==
  x1 : Inport
  x2 : Inport  Port=2
  x6 : Inport  Port=3
  Cos : Trigonometry  Operator=cos
  Product1 : Product  Inputs=3
  Tan : Trigonometry  Operator=tan
  x6cos(x1)tan(x2) : Outport
  wires:
  x6/1 -> Product1/3
  x1/1 -> Cos/1
  Cos/1 -> Product1/1
  x2/1 -> Tan/1
  Product1/1 -> x6cos(x1)tan(x2)/1
  Tan/1 -> Product1/2

== system Quadcopter_nonlinear/Quadcopter 3DOF Nonlinear System7/Quad System1/Quad System/dot(x2)/1/Subsystem ==
  x1 : Inport
  x5 : Inport  Port=2
  Cos : Trigonometry  Operator=cos
  Product : Product
  Out1 : Outport
  wires:
  Cos/1 -> Product/1
  Product/1 -> Out1/1
  x1/1 -> Cos/1
  x5/1 -> Product/2

== system Quadcopter_nonlinear/Quadcopter 3DOF Nonlinear System7/Quad System1/Quad System/dot(x2)/Subsystem/Subsystem1 ==
  x1 : Inport
  x6 : Inport  Port=2
  Product1 : Product
  Sin : Trigonometry
  Out1 : Outport
  wires:
  x6/1 -> Product1/2
  x1/1 -> Sin/1
  Sin/1 -> Product1/1
  Product1/1 -> Out1/1

== system Quadcopter_nonlinear/Quadcopter 3DOF Nonlinear System7/Quad System1/Quad System/dot(x3)/1/Subsystem ==
  x1 : Inport
  x5 : Inport  Port=2
  Product : Product
  Sin : Trigonometry
  x5sin(x1) : Outport
  wires:
  Sin/1 -> Product/1
  Product/1 -> x5sin(x1)/1
  x1/1 -> Sin/1
  x5/1 -> Product/2

== system Quadcopter_nonlinear/Quadcopter 3DOF Nonlinear System7/Quad System1/Quad System/dot(x3)/Subsystem/Subsystem1 ==
  x1 : Inport
  x6 : Inport  Port=2
  Cos : Trigonometry  Operator=cos
  Product1 : Product
  Out1 : Outport
  wires:
  x6/1 -> Product1/2
  x1/1 -> Cos/1
  Cos/1 -> Product1/1
  Product1/1 -> Out1/1

== system Quadcopter_nonlinear/Quadcopter 3DOF Nonlinear System7/Quad System1/Quad System/dot(x3)/Subsystem1/Sec ==
  x2 : Inport
  Constant : Constant
  Cos : Trigonometry  Operator=cos
  Divide : Product  Inputs=*/
  Sec(x2) : Outport
  wires:
  Constant/1 -> Divide/1
  Cos/1 -> Divide/2
  Divide/1 -> Sec(x2)/1
  x2/1 -> Cos/1

== system Quadcopter_nonlinear/Quadcopter 3DOF Nonlinear System8/Quad System1/Quad System/dot(x1)/1/Subsystem ==
  x1 : Inport
  x2 : Inport  Port=2
  x5 : Inport  Port=3
  Product : Product  Inputs=3
  Sin : Trigonometry
  Tan : Trigonometry  Operator=tan
  x5sin(x1)tan(x2) : Outport
  wires:
  Sin/1 -> Product/1
  x5/1 -> Product/3
  Product/1 -> x5sin(x1)tan(x2)/1
  x1/1 -> Sin/1
  x2/1 -> Tan/1
  Tan/1 -> Product/2

== system Quadcopter_nonlinear/Quadcopter 3DOF Nonlinear System8/Quad System1/Quad System/dot(x1)/Subsystem/Subsystem1 ==
  x1 : Inport
  x2 : Inport  Port=2
  x6 : Inport  Port=3
  Cos : Trigonometry  Operator=cos
  Product1 : Product  Inputs=3
  Tan : Trigonometry  Operator=tan
  x6cos(x1)tan(x2) : Outport
  wires:
  x6/1 -> Product1/3
  x1/1 -> Cos/1
  Cos/1 -> Product1/1
  x2/1 -> Tan/1
  Product1/1 -> x6cos(x1)tan(x2)/1
  Tan/1 -> Product1/2

== system Quadcopter_nonlinear/Quadcopter 3DOF Nonlinear System8/Quad System1/Quad System/dot(x2)/1/Subsystem ==
  x1 : Inport
  x5 : Inport  Port=2
  Cos : Trigonometry  Operator=cos
  Product : Product
  Out1 : Outport
  wires:
  Cos/1 -> Product/1
  Product/1 -> Out1/1
  x1/1 -> Cos/1
  x5/1 -> Product/2

== system Quadcopter_nonlinear/Quadcopter 3DOF Nonlinear System8/Quad System1/Quad System/dot(x2)/Subsystem/Subsystem1 ==
  x1 : Inport
  x6 : Inport  Port=2
  Product1 : Product
  Sin : Trigonometry
  Out1 : Outport
  wires:
  x6/1 -> Product1/2
  x1/1 -> Sin/1
  Sin/1 -> Product1/1
  Product1/1 -> Out1/1

== system Quadcopter_nonlinear/Quadcopter 3DOF Nonlinear System8/Quad System1/Quad System/dot(x3)/1/Subsystem ==
  x1 : Inport
  x5 : Inport  Port=2
  Product : Product
  Sin : Trigonometry
  x5sin(x1) : Outport
  wires:
  Sin/1 -> Product/1
  Product/1 -> x5sin(x1)/1
  x1/1 -> Sin/1
  x5/1 -> Product/2

== system Quadcopter_nonlinear/Quadcopter 3DOF Nonlinear System8/Quad System1/Quad System/dot(x3)/Subsystem/Subsystem1 ==
  x1 : Inport
  x6 : Inport  Port=2
  Cos : Trigonometry  Operator=cos
  Product1 : Product
  Out1 : Outport
  wires:
  x6/1 -> Product1/2
  x1/1 -> Cos/1
  Cos/1 -> Product1/1
  Product1/1 -> Out1/1

== system Quadcopter_nonlinear/Quadcopter 3DOF Nonlinear System8/Quad System1/Quad System/dot(x3)/Subsystem1/Sec ==
  x2 : Inport
  Constant : Constant
  Cos : Trigonometry  Operator=cos
  Divide : Product  Inputs=*/
  Sec(x2) : Outport
  wires:
  Constant/1 -> Divide/1
  Cos/1 -> Divide/2
  Divide/1 -> Sec(x2)/1
  x2/1 -> Cos/1

== system Quadcopter_nonlinear/Quadcopter 3DOF Nonlinear System9/Quad System1/Quad System/dot(x1)/1/Subsystem ==
  x1 : Inport
  x2 : Inport  Port=2
  x5 : Inport  Port=3
  Product : Product  Inputs=3
  Sin : Trigonometry
  Tan : Trigonometry  Operator=tan
  x5sin(x1)tan(x2) : Outport
  wires:
  Sin/1 -> Product/1
  x5/1 -> Product/3
  Product/1 -> x5sin(x1)tan(x2)/1
  x1/1 -> Sin/1
  x2/1 -> Tan/1
  Tan/1 -> Product/2

== system Quadcopter_nonlinear/Quadcopter 3DOF Nonlinear System9/Quad System1/Quad System/dot(x1)/Subsystem/Subsystem1 ==
  x1 : Inport
  x2 : Inport  Port=2
  x6 : Inport  Port=3
  Cos : Trigonometry  Operator=cos
  Product1 : Product  Inputs=3
  Tan : Trigonometry  Operator=tan
  x6cos(x1)tan(x2) : Outport
  wires:
  x6/1 -> Product1/3
  x1/1 -> Cos/1
  Cos/1 -> Product1/1
  x2/1 -> Tan/1
  Product1/1 -> x6cos(x1)tan(x2)/1
  Tan/1 -> Product1/2

== system Quadcopter_nonlinear/Quadcopter 3DOF Nonlinear System9/Quad System1/Quad System/dot(x2)/1/Subsystem ==
  x1 : Inport
  x5 : Inport  Port=2
  Cos : Trigonometry  Operator=cos
  Product : Product
  Out1 : Outport
  wires:
  Cos/1 -> Product/1
  Product/1 -> Out1/1
  x1/1 -> Cos/1
  x5/1 -> Product/2

== system Quadcopter_nonlinear/Quadcopter 3DOF Nonlinear System9/Quad System1/Quad System/dot(x2)/Subsystem/Subsystem1 ==
  x1 : Inport
  x6 : Inport  Port=2
  Product1 : Product
  Sin : Trigonometry
  Out1 : Outport
  wires:
  x6/1 -> Product1/2
  x1/1 -> Sin/1
  Sin/1 -> Product1/1
  Product1/1 -> Out1/1

== system Quadcopter_nonlinear/Quadcopter 3DOF Nonlinear System9/Quad System1/Quad System/dot(x3)/1/Subsystem ==
  x1 : Inport
  x5 : Inport  Port=2
  Product : Product
  Sin : Trigonometry
  x5sin(x1) : Outport
  wires:
  Sin/1 -> Product/1
  Product/1 -> x5sin(x1)/1
  x1/1 -> Sin/1
  x5/1 -> Product/2

== system Quadcopter_nonlinear/Quadcopter 3DOF Nonlinear System9/Quad System1/Quad System/dot(x3)/Subsystem/Subsystem1 ==
  x1 : Inport
  x6 : Inport  Port=2
  Cos : Trigonometry  Operator=cos
  Product1 : Product
  Out1 : Outport
  wires:
  x6/1 -> Product1/2
  x1/1 -> Cos/1
  Cos/1 -> Product1/1
  Product1/1 -> Out1/1

== system Quadcopter_nonlinear/Quadcopter 3DOF Nonlinear System9/Quad System1/Quad System/dot(x3)/Subsystem1/Sec ==
  x2 : Inport
  Constant : Constant
  Cos : Trigonometry  Operator=cos
  Divide : Product  Inputs=*/
  Sec(x2) : Outport
  wires:
  Constant/1 -> Divide/1
  Cos/1 -> Divide/2
  Divide/1 -> Sec(x2)/1
  x2/1 -> Cos/1

== matlab function Quadcopter_nonlinear/Quadcopter 3DOF Nonlinear System4/Quad System1/Quad System/MATLAB Function ==
  data: omega input; u output; b input; d input; d_cg input
function u = fcn(omega, b, d, d_cg)

u = zeros(1, 3);

u(1) = b*d_cg*(omega(2)^2 - omega(4)^2); % l
u(2) = b*d_cg*(omega(1)^2 - omega(3)^2); % m
u(3) = d*(omega(1)^2 - omega(2)^2 + omega(3)^2 - omega(4)^2); % n

== matlab function Quadcopter_nonlinear/Quadcopter 3DOF Nonlinear System4/Quad System1/Quad System/MATLAB Function1 ==
  data: X input; omega input; dot_x4 output; u input; Gamma input; dot_x5 output; dot_x6 output
function [dot_x4, dot_x5, dot_x6]  = fcn(X, omega, u, Gamma)



l = u(1);
m = u(2);
n = u(3);

p = X(4);
q = X(5);
r = X(6);

Gamma1 = Gamma(1);
Gamma2 = Gamma(2);
Gamma3 = Gamma(3);
Gamma4 = Gamma(4);
Gamma5 = Gamma(5);
Gamma6 = Gamma(6);
Gamma7 = Gamma(7);
Gamma8 = Gamma(8);
Gamma9 = Gamma(9);
Gamma10 = Gamma(10);
Gamma11 = Gamma(11);

Omega_r = -omega(1) + omega(2) - omega(3) + omega(4);

dot_x4 = Gamma1*p*q - Gamma2*q*r + Gamma3*l + Gamma4*n + Gamma5*Omega_r;
dot_x5 = Gamma6*p*r - Gamma7*(p^2-r^2) + Gamma8*m + Gamma9*Omega_r;
dot_x6 = Gamma10*p*q - Gamma1*q*r + Gamma4*l + Gamma11*n;

== matlab function Quadcopter_nonlinear/Quadcopter 3DOF Nonlinear System1/Quad System1/Quad System/MATLAB Function ==
  data: omega input; u output; b input; d input; d_cg input
function u = fcn(omega, b, d, d_cg)

u = zeros(1, 3);

u(1) = b*d_cg*(omega(2)^2 - omega(4)^2); % l
u(2) = b*d_cg*(omega(1)^2 - omega(3)^2); % m
u(3) = d*(omega(1)^2 - omega(2)^2 + omega(3)^2 - omega(4)^2); % n

== matlab function Quadcopter_nonlinear/Quadcopter 3DOF Nonlinear System5/Quad System1/Quad System/MATLAB Function ==
  data: omega input; u output; b input; d input; d_cg input
function u = fcn(omega, b, d, d_cg)

u = zeros(1, 3);

u(1) = b*d_cg*(omega(2)^2 - omega(4)^2); % l
u(2) = b*d_cg*(omega(1)^2 - omega(3)^2); % m
u(3) = d*(omega(1)^2 - omega(2)^2 + omega(3)^2 - omega(4)^2); % n

== matlab function Quadcopter_nonlinear/Quadcopter 3DOF Nonlinear System5/Quad System1/Quad System/MATLAB Function1 ==
  data: X input; omega input; dot_x4 output; u input; Gamma input; dot_x5 output; dot_x6 output
function [dot_x4, dot_x5, dot_x6]  = fcn(X, omega, u, Gamma)



l = u(1);
m = u(2);
n = u(3);

p = X(4);
q = X(5);
r = X(6);

Gamma1 = Gamma(1);
Gamma2 = Gamma(2);
Gamma3 = Gamma(3);
Gamma4 = Gamma(4);
Gamma5 = Gamma(5);
Gamma6 = Gamma(6);
Gamma7 = Gamma(7);
Gamma8 = Gamma(8);
Gamma9 = Gamma(9);
Gamma10 = Gamma(10);
Gamma11 = Gamma(11);

Omega_r = -omega(1) + omega(2) - omega(3) + omega(4);

dot_x4 = Gamma1*p*q - Gamma2*q*r + Gamma3*l + Gamma4*n + Gamma5*Omega_r;
dot_x5 = Gamma6*p*r - Gamma7*(p^2-r^2) + Gamma8*m + Gamma9*Omega_r;
dot_x6 = Gamma10*p*q - Gamma1*q*r + Gamma4*l + Gamma11*n;

== matlab function Quadcopter_nonlinear/Quadcopter 3DOF Nonlinear System6/Quad System1/Quad System/MATLAB Function ==
  data: omega input; u output; b input; d input; d_cg input
function u = fcn(omega, b, d, d_cg)

u = zeros(1, 3);

u(1) = b*d_cg*(omega(2)^2 - omega(4)^2); % l
u(2) = b*d_cg*(omega(1)^2 - omega(3)^2); % m
u(3) = d*(omega(1)^2 - omega(2)^2 + omega(3)^2 - omega(4)^2); % n

== matlab function Quadcopter_nonlinear/Quadcopter 3DOF Nonlinear System6/Quad System1/Quad System/MATLAB Function1 ==
  data: X input; omega input; dot_x4 output; u input; Gamma input; dot_x5 output; dot_x6 output
function [dot_x4, dot_x5, dot_x6]  = fcn(X, omega, u, Gamma)



l = u(1);
m = u(2);
n = u(3);

p = X(4);
q = X(5);
r = X(6);

Gamma1 = Gamma(1);
Gamma2 = Gamma(2);
Gamma3 = Gamma(3);
Gamma4 = Gamma(4);
Gamma5 = Gamma(5);
Gamma6 = Gamma(6);
Gamma7 = Gamma(7);
Gamma8 = Gamma(8);
Gamma9 = Gamma(9);
Gamma10 = Gamma(10);
Gamma11 = Gamma(11);

Omega_r = -omega(1) + omega(2) - omega(3) + omega(4);

dot_x4 = Gamma1*p*q - Gamma2*q*r + Gamma3*l + Gamma4*n + Gamma5*Omega_r;
dot_x5 = Gamma6*p*r - Gamma7*(p^2-r^2) + Gamma8*m + Gamma9*Omega_r;
dot_x6 = Gamma10*p*q - Gamma1*q*r + Gamma4*l + Gamma11*n;

== matlab function Quadcopter_nonlinear/Quadcopter 3DOF Nonlinear System7/Quad System1/Quad System/MATLAB Function ==
  data: omega input; u output; b input; d input; d_cg input
function u = fcn(omega, b, d, d_cg)

u = zeros(1, 3);

u(1) = b*d_cg*(omega(2)^2 - omega(4)^2); % l
u(2) = b*d_cg*(omega(1)^2 - omega(3)^2); % m
u(3) = d*(omega(1)^2 - omega(2)^2 + omega(3)^2 - omega(4)^2); % n

== matlab function Quadcopter_nonlinear/Quadcopter 3DOF Nonlinear System7/Quad System1/Quad System/MATLAB Function1 ==
  data: X input; omega input; dot_x4 output; u input; Gamma input; dot_x5 output; dot_x6 output
function [dot_x4, dot_x5, dot_x6]  = fcn(X, omega, u, Gamma)



l = u(1);
m = u(2);
n = u(3);

p = X(4);
q = X(5);
r = X(6);

Gamma1 = Gamma(1);
Gamma2 = Gamma(2);
Gamma3 = Gamma(3);
Gamma4 = Gamma(4);
Gamma5 = Gamma(5);
Gamma6 = Gamma(6);
Gamma7 = Gamma(7);
Gamma8 = Gamma(8);
Gamma9 = Gamma(9);
Gamma10 = Gamma(10);
Gamma11 = Gamma(11);

Omega_r = -omega(1) + omega(2) - omega(3) + omega(4);

dot_x4 = Gamma1*p*q - Gamma2*q*r + Gamma3*l + Gamma4*n + Gamma5*Omega_r;
dot_x5 = Gamma6*p*r - Gamma7*(p^2-r^2) + Gamma8*m + Gamma9*Omega_r;
dot_x6 = Gamma10*p*q - Gamma1*q*r + Gamma4*l + Gamma11*n;

== matlab function Quadcopter_nonlinear/Quadcopter 3DOF Nonlinear System8/Quad System1/Quad System/MATLAB Function ==
  data: omega input; u output; b input; d input; d_cg input
function u = fcn(omega, b, d, d_cg)

u = zeros(1, 3);

u(1) = b*d_cg*(omega(2)^2 - omega(4)^2); % l
u(2) = b*d_cg*(omega(1)^2 - omega(3)^2); % m
u(3) = d*(omega(1)^2 - omega(2)^2 + omega(3)^2 - omega(4)^2); % n

== matlab function Quadcopter_nonlinear/Quadcopter 3DOF Nonlinear System8/Quad System1/Quad System/MATLAB Function1 ==
  data: X input; omega input; dot_x4 output; u input; Gamma input; dot_x5 output; dot_x6 output
function [dot_x4, dot_x5, dot_x6]  = fcn(X, omega, u, Gamma)



l = u(1);
m = u(2);
n = u(3);

p = X(4);
q = X(5);
r = X(6);

Gamma1 = Gamma(1);
Gamma2 = Gamma(2);
Gamma3 = Gamma(3);
Gamma4 = Gamma(4);
Gamma5 = Gamma(5);
Gamma6 = Gamma(6);
Gamma7 = Gamma(7);
Gamma8 = Gamma(8);
Gamma9 = Gamma(9);
Gamma10 = Gamma(10);
Gamma11 = Gamma(11);

Omega_r = -omega(1) + omega(2) - omega(3) + omega(4);

dot_x4 = Gamma1*p*q - Gamma2*q*r + Gamma3*l + Gamma4*n + Gamma5*Omega_r;
dot_x5 = Gamma6*p*r - Gamma7*(p^2-r^2) + Gamma8*m + Gamma9*Omega_r;
dot_x6 = Gamma10*p*q - Gamma1*q*r + Gamma4*l + Gamma11*n;

== matlab function Quadcopter_nonlinear/Quadcopter 3DOF Nonlinear System9/Quad System1/Quad System/MATLAB Function ==
  data: omega input; u output; b input; d input; d_cg input
function u = fcn(omega, b, d, d_cg)

u = zeros(1, 3);

u(1) = b*d_cg*(omega(2)^2 - omega(4)^2); % l
u(2) = b*d_cg*(omega(1)^2 - omega(3)^2); % m
u(3) = d*(omega(1)^2 - omega(2)^2 + omega(3)^2 - omega(4)^2); % n

== matlab function Quadcopter_nonlinear/Quadcopter 3DOF Nonlinear System/Quad System1/Quad System/MATLAB Function ==
  data: omega input; u output; b input; d input; d_cg input
function u = fcn(omega, b, d, d_cg)

u = zeros(1, 3);

u(1) = b*d_cg*(omega(2)^2 - omega(4)^2); % l
u(2) = b*d_cg*(omega(1)^2 - omega(3)^2); % m
u(3) = d*(omega(1)^2 - omega(2)^2 + omega(3)^2 - omega(4)^2); % n

== matlab function Quadcopter_nonlinear/Quadcopter 3DOF Nonlinear System9/Quad System1/Quad System/MATLAB Function1 ==
  data: X input; omega input; dot_x4 output; u input; Gamma input; dot_x5 output; dot_x6 output
function [dot_x4, dot_x5, dot_x6]  = fcn(X, omega, u, Gamma)



l = u(1);
m = u(2);
n = u(3);

p = X(4);
q = X(5);
r = X(6);

Gamma1 = Gamma(1);
Gamma2 = Gamma(2);
Gamma3 = Gamma(3);
Gamma4 = Gamma(4);
Gamma5 = Gamma(5);
Gamma6 = Gamma(6);
Gamma7 = Gamma(7);
Gamma8 = Gamma(8);
Gamma9 = Gamma(9);
Gamma10 = Gamma(10);
Gamma11 = Gamma(11);

Omega_r = -omega(1) + omega(2) - omega(3) + omega(4);

dot_x4 = Gamma1*p*q - Gamma2*q*r + Gamma3*l + Gamma4*n + Gamma5*Omega_r;
dot_x5 = Gamma6*p*r - Gamma7*(p^2-r^2) + Gamma8*m + Gamma9*Omega_r;
dot_x6 = Gamma10*p*q - Gamma1*q*r + Gamma4*l + Gamma11*n;

== matlab function Quadcopter_nonlinear/Quadcopter 3DOF Nonlinear System/Quad System1/Quad System/MATLAB Function1 ==
  data: X input; omega input; dot_x4 output; u input; Gamma input; dot_x5 output; dot_x6 output
function [dot_x4, dot_x5, dot_x6]  = fcn(X, omega, u, Gamma)



l = u(1);
m = u(2);
n = u(3);

p = X(4);
q = X(5);
r = X(6);

Gamma1 = Gamma(1);
Gamma2 = Gamma(2);
Gamma3 = Gamma(3);
Gamma4 = Gamma(4);
Gamma5 = Gamma(5);
Gamma6 = Gamma(6);
Gamma7 = Gamma(7);
Gamma8 = Gamma(8);
Gamma9 = Gamma(9);
Gamma10 = Gamma(10);
Gamma11 = Gamma(11);

Omega_r = -omega(1) + omega(2) - omega(3) + omega(4);

dot_x4 = Gamma1*p*q - Gamma2*q*r + Gamma3*l + Gamma4*n + Gamma5*Omega_r;
dot_x5 = Gamma6*p*r - Gamma7*(p^2-r^2) + Gamma8*m + Gamma9*Omega_r;
dot_x6 = Gamma10*p*q - Gamma1*q*r + Gamma4*l + Gamma11*n;

== matlab function Quadcopter_nonlinear/Quadcopter 3DOF Nonlinear System1/Quad System1/Quad System/MATLAB Function1 ==
  data: X input; omega input; dot_x4 output; u input; Gamma input; dot_x5 output; dot_x6 output
function [dot_x4, dot_x5, dot_x6]  = fcn(X, omega, u, Gamma)



l = u(1);
m = u(2);
n = u(3);

p = X(4);
q = X(5);
r = X(6);

Gamma1 = Gamma(1);
Gamma2 = Gamma(2);
Gamma3 = Gamma(3);
Gamma4 = Gamma(4);
Gamma5 = Gamma(5);
Gamma6 = Gamma(6);
Gamma7 = Gamma(7);
Gamma8 = Gamma(8);
Gamma9 = Gamma(9);
Gamma10 = Gamma(10);
Gamma11 = Gamma(11);

Omega_r = -omega(1) + omega(2) - omega(3) + omega(4);

dot_x4 = Gamma1*p*q - Gamma2*q*r + Gamma3*l + Gamma4*n + Gamma5*Omega_r;
dot_x5 = Gamma6*p*r - Gamma7*(p^2-r^2) + Gamma8*m + Gamma9*Omega_r;
dot_x6 = Gamma10*p*q - Gamma1*q*r + Gamma4*l + Gamma11*n;

== matlab function Quadcopter_nonlinear/Quadcopter 3DOF Nonlinear System2/Quad System1/Quad System/MATLAB Function ==
  data: omega input; u output; b input; d input; d_cg input
function u = fcn(omega, b, d, d_cg)

u = zeros(1, 3);

u(1) = b*d_cg*(omega(2)^2 - omega(4)^2); % l
u(2) = b*d_cg*(omega(1)^2 - omega(3)^2); % m
u(3) = d*(omega(1)^2 - omega(2)^2 + omega(3)^2 - omega(4)^2); % n

== matlab function Quadcopter_nonlinear/Quadcopter 3DOF Nonlinear System2/Quad System1/Quad System/MATLAB Function1 ==
  data: X input; omega input; dot_x4 output; u input; Gamma input; dot_x5 output; dot_x6 output
function [dot_x4, dot_x5, dot_x6]  = fcn(X, omega, u, Gamma)



l = u(1);
m = u(2);
n = u(3);

p = X(4);
q = X(5);
r = X(6);

Gamma1 = Gamma(1);
Gamma2 = Gamma(2);
Gamma3 = Gamma(3);
Gamma4 = Gamma(4);
Gamma5 = Gamma(5);
Gamma6 = Gamma(6);
Gamma7 = Gamma(7);
Gamma8 = Gamma(8);
Gamma9 = Gamma(9);
Gamma10 = Gamma(10);
Gamma11 = Gamma(11);

Omega_r = -omega(1) + omega(2) - omega(3) + omega(4);

dot_x4 = Gamma1*p*q - Gamma2*q*r + Gamma3*l + Gamma4*n + Gamma5*Omega_r;
dot_x5 = Gamma6*p*r - Gamma7*(p^2-r^2) + Gamma8*m + Gamma9*Omega_r;
dot_x6 = Gamma10*p*q - Gamma1*q*r + Gamma4*l + Gamma11*n;

== matlab function Quadcopter_nonlinear/Quadcopter 3DOF Nonlinear System3/Quad System1/Quad System/MATLAB Function ==
  data: omega input; u output; b input; d input; d_cg input
function u = fcn(omega, b, d, d_cg)

u = zeros(1, 3);

u(1) = b*d_cg*(omega(2)^2 - omega(4)^2); % l
u(2) = b*d_cg*(omega(1)^2 - omega(3)^2); % m
u(3) = d*(omega(1)^2 - omega(2)^2 + omega(3)^2 - omega(4)^2); % n

== matlab function Quadcopter_nonlinear/Quadcopter 3DOF Nonlinear System3/Quad System1/Quad System/MATLAB Function1 ==
  data: X input; omega input; dot_x4 output; u input; Gamma input; dot_x5 output; dot_x6 output
function [dot_x4, dot_x5, dot_x6]  = fcn(X, omega, u, Gamma)



l = u(1);
m = u(2);
n = u(3);

p = X(4);
q = X(5);
r = X(6);

Gamma1 = Gamma(1);
Gamma2 = Gamma(2);
Gamma3 = Gamma(3);
Gamma4 = Gamma(4);
Gamma5 = Gamma(5);
Gamma6 = Gamma(6);
Gamma7 = Gamma(7);
Gamma8 = Gamma(8);
Gamma9 = Gamma(9);
Gamma10 = Gamma(10);
Gamma11 = Gamma(11);

Omega_r = -omega(1) + omega(2) - omega(3) + omega(4);

dot_x4 = Gamma1*p*q - Gamma2*q*r + Gamma3*l + Gamma4*n + Gamma5*Omega_r;
dot_x5 = Gamma6*p*r - Gamma7*(p^2-r^2) + Gamma8*m + Gamma9*Omega_r;
dot_x6 = Gamma10*p*q - Gamma1*q*r + Gamma4*l + Gamma11*n;
